simulink model "B_10"  (R2018b)
settings: Solver=VariableStepAuto  StartTime=0.0  StopTime=1  MaxStep=1e-4  RelTol=1e-6
StopFcn:
  | %CELEC_plot;
libraries: fuzblock x1
settings Model: Creator=Administrator  LastModifiedBy=Administrator

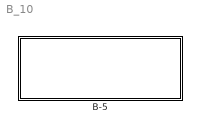
== system B_10 ==
  B-5 : Subsystem  mask{Vset=10, R=2, L=0.02, J=10, KE=1.8, KT=17.2}
      mask prompts: Vset "电源电压(V)"; R "电枢电阻(Ω）"; L "电枢电感(H)"; J "转动惯量(kg.m^3)"; KE "反电势系数(V/rpm)"; KT "电磁转矩系数(N.m/A)"

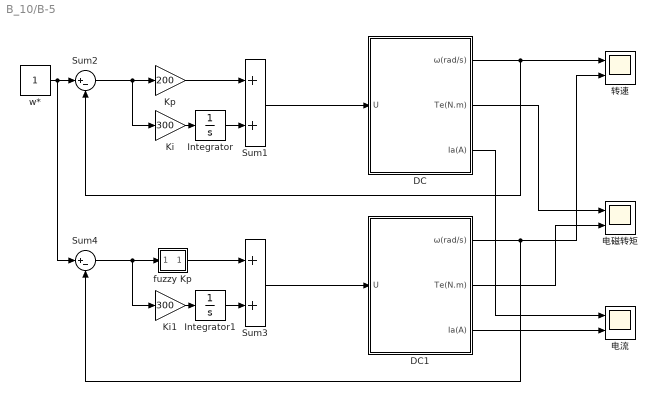
== system B_10/B-5 ==
  DC : Subsystem
  DC1 : Subsystem
  Integrator : Integrator
  Integrator1 : Integrator
  Ki : Gain  Gain=300
  Ki1 : Gain  Gain=300
  Kp : Gain  Gain=200
  Sum1 : Sum
  Sum2 : Sum  Inputs=|+-
  Sum3 : Sum
  Sum4 : Sum  Inputs=|+-
  fuzzy Kp : Subsystem
  w* : Constant
  电流 : Scope  NumInputPorts=2
  电磁转矩 : Scope  NumInputPorts=2
  转速 : Scope  NumInputPorts=2
  wires:
  Sum2/1 -> Ki/1, Kp/1
  Kp/1 -> Sum1/1
  Ki/1 -> Integrator/1
  Integrator/1 -> Sum1/2
  w*/1 -> Sum4/1, Sum2/1
  DC/1(ω(rad/s)) -> 转速/1, Sum2/2
  Sum1/1 -> DC/1(U)
  DC/2(Te(N.m)) -> 电磁转矩/1
  DC/3(Ia(A)) -> 电流/1
  Integrator1/1 -> Sum3/2
  Sum3/1 -> DC1/1(U)
  DC1/2(Te(N.m)) -> 电磁转矩/2
  Ki1/1 -> Integrator1/1
  Sum4/1 -> fuzzy Kp/1(" "), Ki1/1
  DC1/1(ω(rad/s)) -> 转速/2, Sum4/2
  DC1/3(Ia(A)) -> 电流/2
  fuzzy Kp/1("  ") -> Sum3/1

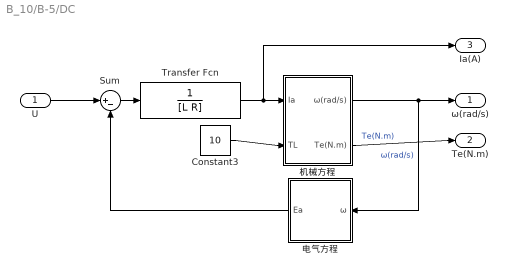
== system B_10/B-5/DC ==
  U : Inport
  Constant3 : Constant  Value=10
  Sum : Sum  Inputs=|+-
  Transfer Fcn : TransferFcn  Denominator=[L R]
  机械方程 : Subsystem
  电气方程 : Subsystem
  ω(rad/s) : Outport
  Te(N.m) : Outport  Port=2
  Ia(A) : Outport  Port=3
  wires:
  Transfer Fcn/1 -> Ia(A)/1, 机械方程/1(Ia)
  Constant3/1 -> 机械方程/2(TL)
  Sum/1 -> Transfer Fcn/1
  机械方程/1(ω(rad/s)) -> 电气方程/1(ω), ω(rad/s)/1  "ω(rad/s)"
  电气方程/1(Ea) -> Sum/2
  U/1 -> Sum/1
  机械方程/2(Te(N.m)) -> Te(N.m)/1  "Te(N.m)"

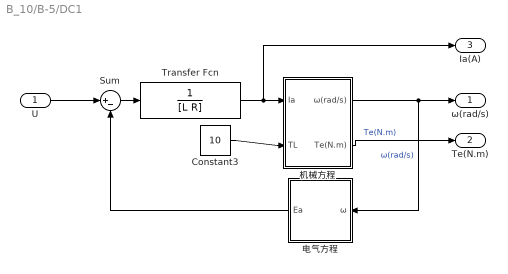
== system B_10/B-5/DC1 ==
  U : Inport
  Constant3 : Constant  Value=10
  Sum : Sum  Inputs=|+-
  Transfer Fcn : TransferFcn  Denominator=[L R]
  机械方程 : Subsystem
  电气方程 : Subsystem
  ω(rad/s) : Outport
  Te(N.m) : Outport  Port=2
  Ia(A) : Outport  Port=3
  wires:
  Transfer Fcn/1 -> Ia(A)/1, 机械方程/1(Ia)
  Constant3/1 -> 机械方程/2(TL)
  Sum/1 -> Transfer Fcn/1
  机械方程/1(ω(rad/s)) -> 电气方程/1(ω), ω(rad/s)/1  "ω(rad/s)"
  电气方程/1(Ea) -> Sum/2
  U/1 -> Sum/1
  机械方程/2(Te(N.m)) -> Te(N.m)/1  "Te(N.m)"

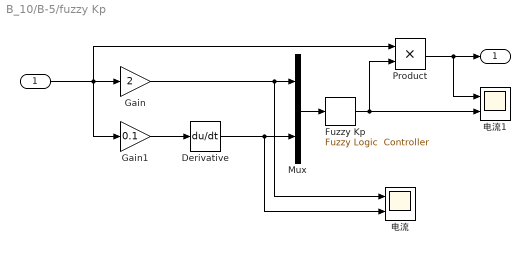
== system B_10/B-5/fuzzy Kp ==
  " " : Inport
  Derivative : Derivative
  Fuzzy Kp : fuzblock/Fuzzy Logic  Controller  FIS=FIS_CELEC  OutputSampleNumber=101  DataType=double  FuzzifiedInputs=off  RuleFiringStrengths=off  RuleOutputs=off  AggregatedOutputs=off  SimulateUsing=Code generation  OutOfRangeInputValueMessage=warning  NoRuleFiredMessage=warning  EmptyOutputFuzzySetMessage=warning
  Gain : Gain  Gain=2
  Gain1 : Gain  Gain=0.1
  Mux : Mux  Inputs=2
  Product : Product
  电流 : Scope  NumInputPorts=2
  电流1 : Scope  NumInputPorts=2
  "  " : Outport
  wires:
  Fuzzy Kp/1 -> 电流1/2, Product/2
  Mux/1 -> Fuzzy Kp/1
  " "/1 -> Product/1, Gain1/1, Gain/1
  Derivative/1 -> 电流/2, Mux/2
  Gain1/1 -> Derivative/1
  Gain/1 -> 电流/1, Mux/1
  Product/1 -> 电流1/1, "  "/1

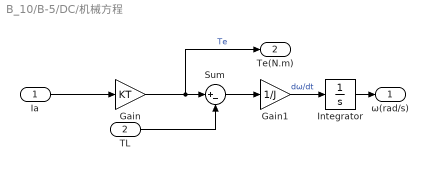
== system B_10/B-5/DC/机械方程 ==
  Ia : Inport
  TL : Inport  Port=2
  Gain : Gain  Gain=KT
  Gain1 : Gain  Gain=1/J
  Integrator : Integrator
  Sum : Sum  Inputs=|+-
  ω(rad/s) : Outport
  Te(N.m) : Outport  Port=2
  wires:
  Gain1/1 -> Integrator/1  "dω/dt"
  Sum/1 -> Gain1/1
  Gain/1 -> Te(N.m)/1, Sum/1  "Te"
  TL/1 -> Sum/2
  Ia/1 -> Gain/1
  Integrator/1 -> ω(rad/s)/1

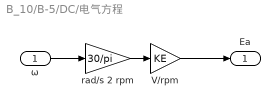
== system B_10/B-5/DC/电气方程 ==
  ω : Inport
  V/rpm : Gain  Gain=KE
  rad/s 2 rpm : Gain  Gain=30/pi
  Ea : Outport
  wires:
  rad/s 2 rpm/1 -> V/rpm/1
  ω/1 -> rad/s 2 rpm/1
  V/rpm/1 -> Ea/1

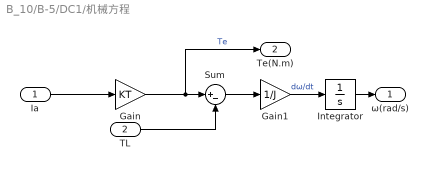
== system B_10/B-5/DC1/机械方程 ==
  Ia : Inport
  TL : Inport  Port=2
  Gain : Gain  Gain=KT
  Gain1 : Gain  Gain=1/J
  Integrator : Integrator
  Sum : Sum  Inputs=|+-
  ω(rad/s) : Outport
  Te(N.m) : Outport  Port=2
  wires:
  Gain1/1 -> Integrator/1  "dω/dt"
  Sum/1 -> Gain1/1
  Gain/1 -> Te(N.m)/1, Sum/1  "Te"
  TL/1 -> Sum/2
  Ia/1 -> Gain/1
  Integrator/1 -> ω(rad/s)/1

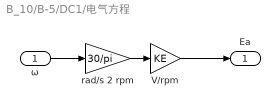
== system B_10/B-5/DC1/电气方程 ==
  ω : Inport
  V/rpm : Gain  Gain=KE
  rad/s 2 rpm : Gain  Gain=30/pi
  Ea : Outport
  wires:
  rad/s 2 rpm/1 -> V/rpm/1
  ω/1 -> rad/s 2 rpm/1
  V/rpm/1 -> Ea/1
